simulink model "blumentopf"  (R2014b)
settings: Solver=ode45  StartTime=0.0  StopTime=10.0  RelTol=1e-3
settings Model: Creator=sigurd  LastModifiedBy=sigurd

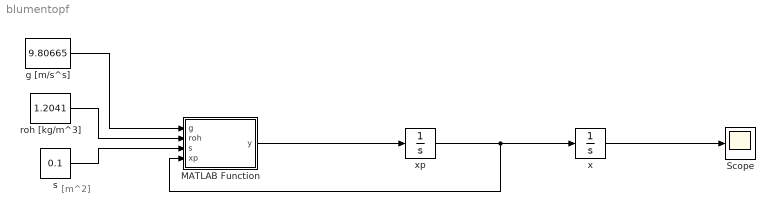
== system blumentopf ==
  note: [m^2]
  MATLAB Function : MATLAB Function  TreatAsAtomicUnit=on
  Scope : Scope
  g [m/s^s] : Constant  Value=9.80665
  roh [kg/m^3] : Constant  Value=1.2041
  s : Constant  Value=0.1
  x : Integrator  InitialCondition=120
  xp : Integrator
  wires:
  xp/1 -> MATLAB Function/4(xp), x/1
  x/1 -> Scope/1
  g [m/s^s]/1 -> MATLAB Function/1(g)
  roh [kg/m^3]/1 -> MATLAB Function/2(roh)
  s/1 -> MATLAB Function/3(s)
  MATLAB Function/1(y) -> xp/1

== matlab function blumentopf/MATLAB Function ==
  data: g input; y output; roh input; s input; xp input
function y = fcn(g,roh,s,xp)
y = -g + (0.5 * roh * s * (xp * xp));
